simulink model "Q6_FIR"  (R2020b)
settings: Solver=VariableStepAuto  StartTime=0.0  StopTime=10.0  RelTol=1e-3
libraries: simulink x1
settings Model: Creator=mluser  LastModifiedBy=mluser

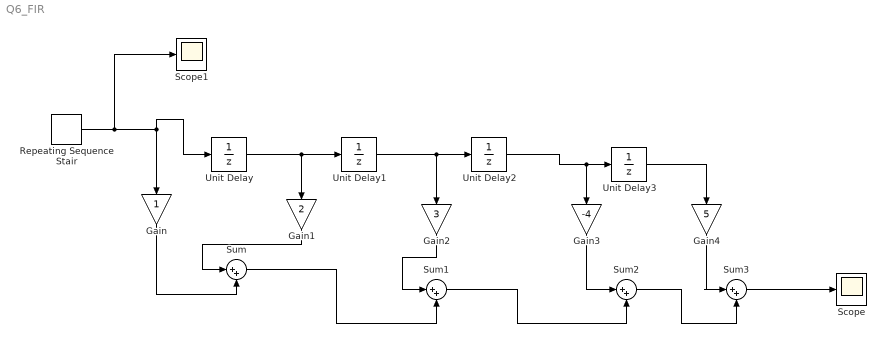
== system Q6_FIR ==
  Gain : Gain
  Gain1 : Gain  Gain=2
  Gain2 : Gain  Gain=3
  Gain3 : Gain  Gain=-4
  Gain4 : Gain  Gain=5
  Repeating Sequence Stair : simulink/Sources/Repeating Sequence Stair  OutValues=[10111].'  tsamp=-1  OutMin=[]  OutMax=[]  OutDataTypeStr=double  OutputDataTypeScalingMode=double  OutDataType=fixdt(0,8)  ConRadixGroup=Best Precision: Vector-wise  OutScaling=2^-12
  Scope : Scope
  Scope1 : Scope
  Sum{,1..3} (4 alike) : Sum  Inputs=|++
  Unit Delay{,1..3} (4 alike) : UnitDelay  SampleTime=-1  HasFrameUpgradeWarning=on
  wires:
  Unit Delay/1 -> Gain1/1, Unit Delay1/1
  Gain1/1 -> Sum/1
  Gain/1 -> Sum/2
  Repeating Sequence Stair/1 -> Scope1/1, Gain/1, Unit Delay/1
  Unit Delay1/1 -> Gain2/1, Unit Delay2/1
  Sum/1 -> Sum1/2
  Gain2/1 -> Sum1/1
  Unit Delay2/1 -> Gain3/1, Unit Delay3/1
  Gain3/1 -> Sum2/1
  Sum1/1 -> Sum2/2
  Sum2/1 -> Sum3/2
  Unit Delay3/1 -> Gain4/1
  Sum3/1 -> Scope/1
  Gain4/1 -> Sum3/1
